simulink library "Detumbling_Controller_lib"  (R2018b)
settings: Solver=VariableStepAuto  StartTime=0.0  StopTime=10.0  RelTol=1e-3
undefined symbols (not defined in the file or in its folder): fswParams
settings Model: Creator=colem  LastModifiedBy=colem

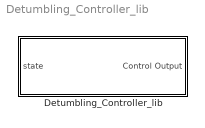
== system Detumbling_Controller_lib ==
  Detumbling_Controller_lib : Subsystem

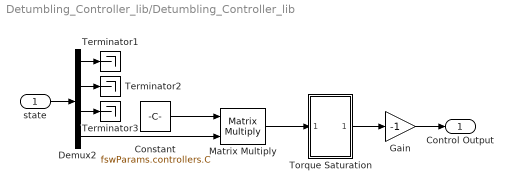
== system Detumbling_Controller_lib/Detumbling_Controller_lib ==
  state : Inport
  Constant : Constant  Value=fswParams.controllers.C
  Demux2 : Demux  Outputs=[3 3 4 3]
  Gain : Gain  Gain=-1
  Matrix Multiply : Product  Multiplication=Matrix(*)
  Terminator1 : Terminator
  Terminator2 : Terminator
  Terminator3 : Terminator
  Torque Saturation : Subsystem
  Control Output : Outport
  wires:
  Constant/1 -> Matrix Multiply/1
  Torque Saturation/1(Out1) -> Gain/1
  Gain/1 -> Control Output/1
  Matrix Multiply/1 -> Torque Saturation/1(In1)
  state/1 -> Demux2/1
  Demux2/1 -> Terminator1/1
  Demux2/2 -> Terminator2/1
  Demux2/3 -> Terminator3/1
  Demux2/4 -> Matrix Multiply/2

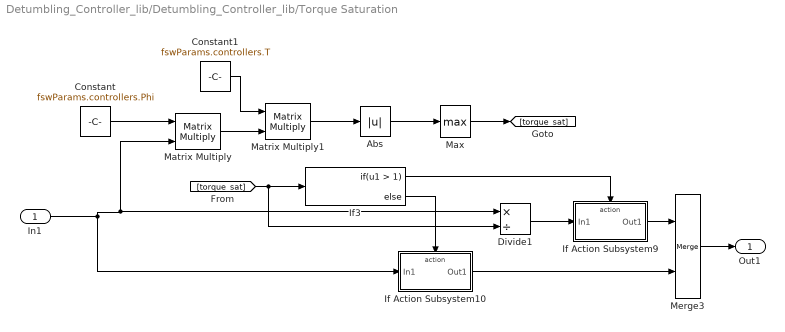
== system Detumbling_Controller_lib/Detumbling_Controller_lib/Torque Saturation ==
  In1 : Inport
  Abs : Abs
  Constant : Constant  Value=fswParams.controllers.Phi
  Constant1 : Constant  Value=fswParams.controllers.T
  Divide1 : Product  Inputs=*/
  If Action Subsystem10 : Subsystem  TreatAsAtomicUnit=on
  If Action Subsystem9 : Subsystem  TreatAsAtomicUnit=on
  If3 : If  IfExpression=u1 > 1
  Matrix Multiply : Product  Multiplication=Matrix(*)
  Matrix Multiply1 : Product  Multiplication=Matrix(*)
  Max : MinMax  Function=max
  Merge3 : Merge
  Out1 : Outport
  wires:
  If Action Subsystem9/1(Out1) -> Merge3/1
  If3/1 -> If Action Subsystem9/Action
  If3/2 -> If Action Subsystem10/Action
  If Action Subsystem10/1(Out1) -> Merge3/2
  Merge3/1 -> Out1/1
  Divide1/1 -> If Action Subsystem9/1(In1)
  Constant/1 -> Matrix Multiply/1
  In1/1 -> Matrix Multiply/2, Divide1/1, If Action Subsystem10/1(In1)
  Matrix Multiply/1 -> Matrix Multiply1/2
  Constant1/1 -> Matrix Multiply1/1
  Matrix Multiply1/1 -> Abs/1
  Abs/1 -> Max/1
  [torque_sat] -> Divide1/2, If3/1
  Max/1 -> [torque_sat]

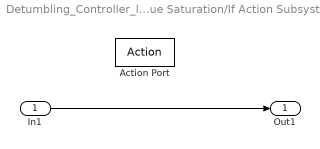
== system Detumbling_Controller_lib/Detumbling_Controller_lib/Torque Saturation/If Action Subsystem10 ==
  In1 : Inport
  Action Port : ActionPort
  Out1 : Outport
  wires:
  In1/1 -> Out1/1

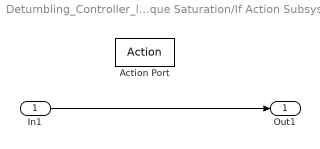
== system Detumbling_Controller_lib/Detumbling_Controller_lib/Torque Saturation/If Action Subsystem9 ==
  In1 : Inport
  Action Port : ActionPort
  Out1 : Outport
  wires:
  In1/1 -> Out1/1
